simulink model "R1_integrator"  (R2014b)
settings: Solver=ode3  SolverMode=SingleTasking  StartTime=0.0  StopTime=Tsim  FixedStep=Ts  RelTol=1e-3
InitFcn:
  | configIntegrator
settings Model: CovMetricSettings=dwe  CovHtmlReporting=off  covSaveCumulativeToWorkspaceVar=off  CovSaveSingleToWorkspaceVar=off  CovExternalEMLEnable=on  CovSFcnEnable=on  Creator=mnade  LastModifiedBy=nina
settings DataIOCC: LimitDataPoints=off  SaveFormat=StructureWithTime
settings DebuggingCC: SolverPrmCheckMsg=none  FrameProcessingCompatibilityMsg=error  SFUnexpectedBacktrackingDiag=error  SFNoUnconditionalDefaultTransitionDiag=error
settings HardwareCC: ProdBitPerPointer=64  ProdLargestAtomicFloat=Float  ProdIntDivRoundTo=Zero  ProdEndianess=LittleEndian  ProdHWDeviceType=Specified
settings ModelReferenceCC: PropagateSignalLabelsOutOfModel=on
settings GRTTargetCC: TargetLangStandard=C99 (ISO)  GeneratePreprocessorConditionals=Use local settings

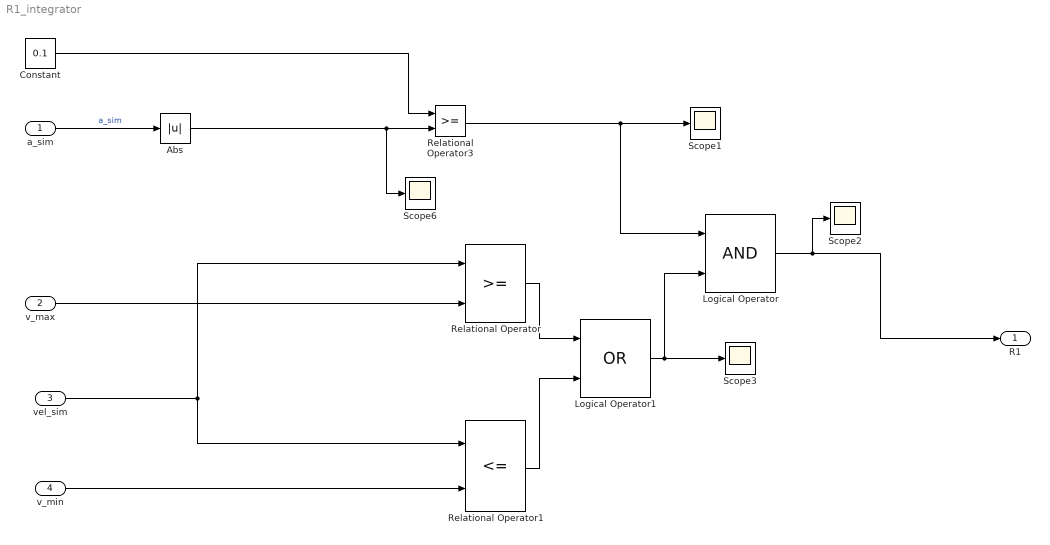
== system R1_integrator ==
  a_sim : Inport
  v_max : Inport  Port=2
  vel_sim : Inport  Port=3
  v_min : Inport  Port=4
  Abs : Abs
  Constant : Constant  Value=0.1
  Logical Operator : Logic  AllPortsSameDT=off  OutDataTypeStr=boolean
  Logical Operator1 : Logic  Operator=OR  AllPortsSameDT=off  OutDataTypeStr=boolean
  Relational Operator : RelationalOperator  OutDataTypeStr=boolean
  Relational Operator1 : RelationalOperator  Operator=<=  OutDataTypeStr=boolean
  Relational Operator3 : RelationalOperator  OutDataTypeStr=boolean
  Scope{1..3,6} (4 alike) : Scope
      Scope3 settings: SaveName=ScopeData3
      Scope6 settings: SaveName=ScopeData5
  R1 : Outport
  wires:
  a_sim/1 -> Abs/1  "a_sim"
  Relational Operator1/1 -> Logical Operator1/2
  Relational Operator/1 -> Logical Operator1/1
  Relational Operator3/1 -> Scope1/1, Logical Operator/1
  Logical Operator1/1 -> Scope3/1, Logical Operator/2
  Constant/1 -> Relational Operator3/1
  v_min/1 -> Relational Operator1/2
  v_max/1 -> Relational Operator/2
  Logical Operator/1 -> Scope2/1, R1/1
  vel_sim/1 -> Relational Operator/1, Relational Operator1/1
  Abs/1 -> Scope6/1, Relational Operator3/2
